simulink model "sl_subsys_fcncallerr5"  (Simulink 7.6)
settings: Solver=FixedStepDiscrete  StartTime=0.0  StopTime=10.0  FixedStep=1  RelTol=1e-3
Description:
  | Ambiguous execution order due to feedback of modified function-call output
  | 
  | The Chart is making the function-call d1=f(), i.e., it is invoking f() and then
  | later using the value d1. When f() executes, it calls g() and attempts to use a
  | modified value of g()'s output, B(g()), thus creating an erroneous model.
settings Model: Creator=The MathWorks Inc.  CovMetricSettings=d  ExtModeAutoUpdateStatusClock=off
settings OptimizationCC: BlockReduction=off  BooleanDataType=off  InlineInvariantSignals=on  InitFltsAndDblsToZero=on
settings DebuggingCC: SaveWithParameterizedLinksMsg=none  SignalResolutionControl=TryResolveAllWithWarning  SolverPrmCheckMsg=none  MultiTaskDSMMsg=warning  MultiTaskCondExecSysMsg=none
settings HardwareCC: TargetUnknown=on
settings SFSimCC: SimParseCustomCode=off
settings RTWCC: IncludeERTFirstTime=on
settings CodeAppCC: CustomSymbolStrFcn=$F$N$M
settings GRTTargetCC: TargetFcnLib=ansi_tfl_tmw.mat

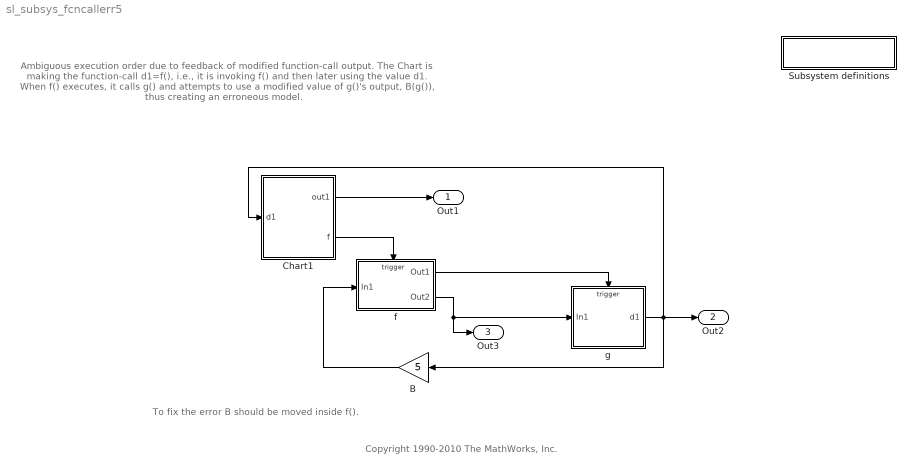
== system sl_subsys_fcncallerr5 ==
  note: Ambiguous execution order due to feedback of modified function-call output.
      |
      | The Chart is making the function-call d1=f(), i.e., it is invoking f() and then
      | later using the value d1. When f() executes, it calls g() and attempts to use a
      | modified value of g()'s output, B(g()), thus creating an erroneous model.
  note: To fix the error B should be moved inside f().
  note: Copyright 1990-2010 The MathWorks, Inc.
  " Subsystem definitions" : Subsystem
      settings: OpenFcn=helpview([matlabroot,'/toolbox/simulink/simdemos/simfeatures/html/sl_subsys_definitions.html']);
      mask Display: disp('Subsystem\ndefinitions')
  B : Gain  Gain=5  SaturateOnIntegerOverflow=on  OutDataTypeStr=Inherit: Same as input  ParamDataTypeStr=Inherit: Same as input
  Chart1 : Stateflow chart  TreatAsAtomicUnit=on
  f : Subsystem  TreatAsAtomicUnit=on
  g : Subsystem  TreatAsAtomicUnit=on
  Out1 : Outport
  Out2 : Outport  Port=2
  Out3 : Outport  Port=3
  wires:
  Chart1/2(f) -> f/Trigger
  f/1(Out1) -> g/Trigger
  f/2(Out2) -> Out3/1, g/1(In1)
  g/1(d1) -> Out2/1, B/1, Chart1/1(d1)
  Chart1/1(out1) -> Out1/1
  B/1 -> f/1(In1)

== system sl_subsys_fcncallerr5/ Subsystem definitions ==

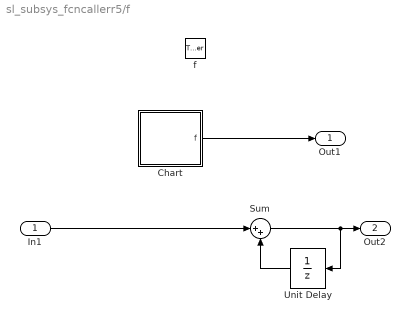
== system sl_subsys_fcncallerr5/f ==
  In1 : Inport
  f : TriggerPort  TriggerType=function-call
  Chart : Stateflow chart  TreatAsAtomicUnit=on
  Sum : Sum  Inputs=|++  SaturateOnIntegerOverflow=on  InputSameDT=on  OutDataTypeStr=Inherit: Same as first input
  Unit Delay : UnitDelay  SampleTime=-1
  Out1 : Outport
  Out2 : Outport  Port=2
  wires:
  Chart/1(f) -> Out1/1
  In1/1 -> Sum/1
  Unit Delay/1 -> Sum/2
  Sum/1 -> Out2/1, Unit Delay/1

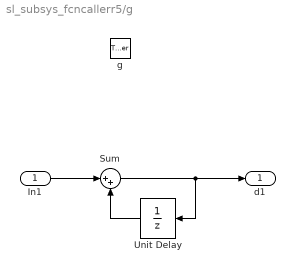
== system sl_subsys_fcncallerr5/g ==
  In1 : Inport
  g : TriggerPort  TriggerType=function-call
  Sum : Sum  Inputs=|++  SaturateOnIntegerOverflow=on  InputSameDT=on  OutDataTypeStr=Inherit: Same as first input
  Unit Delay : UnitDelay  SampleTime=-1
  d1 : Outport
  wires:
  In1/1 -> Sum/1
  Unit Delay/1 -> Sum/2
  Sum/1 -> d1/1, Unit Delay/1

== stateflow chart f/Chart ==
  state one
  state two
  one -> two : /f;
  two -> one : /f;
  (default) -> one
  events: f output FUNCTION_CALL_EVENT

== stateflow chart Chart1 ==
  state one/
    entry:f;out1=d1+5;
  state two/
    entry: f;out1=d1-5;
  one -> two
  two -> one
  (default) -> one
  data: d1 input double; out1 output double; out local double
  events: f output FUNCTION_CALL_EVENT
